simulink model "Bidirectional_Charger_for_EVs"  (R2023a)
settings: Solver=VariableStepAuto  StartTime=0.0  StopTime=0.5  RelTol=1e-3
values from neighbouring files (symbols this model uses):
  fsw = 120e3    (= 120000)    [parametreler_DAB.m]
  Kp = sqrt(fsw*L)    [parametreler_DAB.m]
  L = 20e-6    (= 2e-05)    [parametreler_DAB.m]
  Tsim = tsw    (= 4.16666666667e-06)    [parametreler_DAB.m]
  tsw = 1/2/fsw    (= 4.16666666667e-06)    [parametreler_DAB.m]
undefined symbols (not defined in the file or in its folder): Ion, Lithium
libraries: spsIGBTDiodeLib x12, spsVoltageMeasurementLib x9, spsMosfetLib x8, spsSeriesRLCBranchLib x8, spsDiodeLib x6, spsCurrentMeasurementLib x5, slpidlib x3, simulink x3, simulink_extras x2, spsTriangleGeneratorLib x2, spsBatteryLib x1, spsLinearTransformerLib x1
settings Model: Creator=Berkan  LastModifiedBy=mahgo
settings ModelReferenceCC: EnableRefExpFcnMdlSchedulingChecks=on

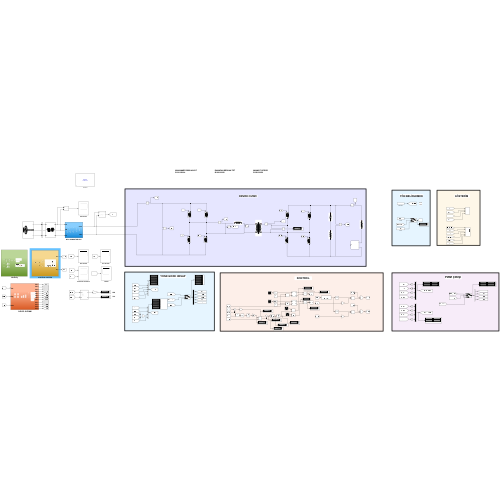
[thumbnail: Simulink's stored preview of the top-level diagram]
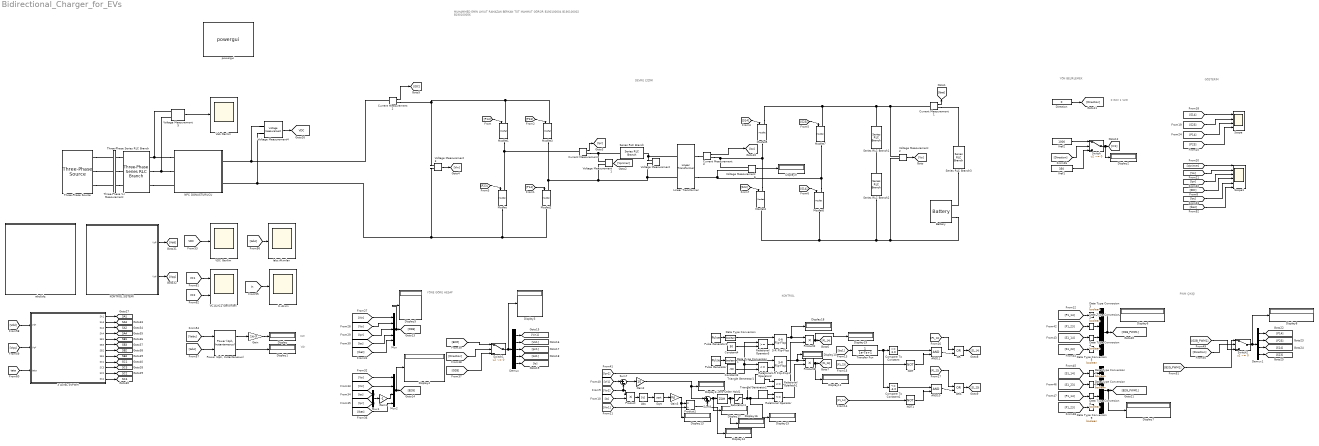
== system Bidirectional_Charger_for_EVs ==
  note: VAr
  note: MUHAMMED EMİN AYKUT RAMAZAN BERKAN TÜT MAHMUT GÖRÜR
      | B190100004 B190100002 B190100056
  note: KW
  note: DEVRE ÇİZİMİ
  note: KONTROL
  note: PWM ÇIKIŞI
  note: 0 G2V
      | 1 V2G
  note: YÖN BELİRLEMEK
  note: GÖSTERİM
  note: YÖNE GÖRE HESAP
  " KONTROL SISTEMI" : Subsystem
  3 LEVEL SVPWM : Subsystem
  AND10 : Logic  IconShape=distinctive  AllPortsSameDT=off  OutDataTypeStr=boolean
  AND11 : Logic  IconShape=distinctive  AllPortsSameDT=off  OutDataTypeStr=boolean
  Abs : Abs  SaturateOnIntegerOverflow=off
  Battery : spsBatteryLib/Battery  BatType=Lithium-Ion  ShowTempParam=off  ThermalPreset=no  ShowAgeParam=off  NomV=350  NomQ=5.4  SOC=0  Batt_Tr=30  PresetModel=on  MaxQ=5.4  MinV=262.5  FullV=407.3955  Dis_rate=2.3478  R=0.64815  Normal_OP=4.8835  expZone="[378.135     0.2653043]"  current=[6.5 13 32.5]  Units=Time  Tci=20  NomT=20  T2=-30  MaxQ2=4.8  FullV2=7.1  Normal_OP2=5.655  expZone2="[6.58           1]"  Rca=0.6  ti=2000  Dp=0  Neq0=0  Tsim=1e6  Ta1=25  Qeol=5.4*0.9  Reol=0.013333*1.2  Char_age=[2.3478, 3]  Dis_age=[2.3478, 10]  N1=1500  N2=10500  N3=1000  N4=1400  Ta2=45  N5=950
  Compare To Constant : simulink/Logic and Bit Operations/Compare To Constant  relop=>=  const=3.0  OutDataTypeStr=boolean
  Compare To Constant1 : simulink/Logic and Bit Operations/Compare To Constant  relop=<=  const=-3.0  OutDataTypeStr=boolean
  Constant3 : Constant  Value=-50
  Constant4 : Constant  Value=50
  Current Measurement{,1..3} (4 alike) : spsCurrentMeasurementLib/Current Measurement  PhasorSimulation=off  OutputType=Complex  PSBequivalent=0
  Data Type Conversion{,1..9} (10 alike) : DataTypeConversion  OutDataTypeStr=boolean  SaturateOnIntegerOverflow=off  RndMeth=Floor
  Demux : Demux  Outputs=5
  Demux1 : Demux
  Direction : Constant  Value=0
  Display{,1..19} (20 alike) : Display
  Gain : Gain  Gain=1e-3
  Gain1 : Gain  Gain=-1
  Gain2 : Gain  Gain=10
  Gain3 : Gain  Gain=Kp
  Iabc Akımları : Scope
  In Akımı : Scope
  Linear Transformer : spsLinearTransformerLib/Linear Transformer  UNITS=SI  NominalPower=[ 250e6 50 ]  winding1=[7.35e+05 4.32 0.45]  winding2=[3.85e+05 4.32 0.45]  ThreeWindings=off  winding3=[3.15e+05 0.7938 6.3169e-05]  RmLm=[1e6 2866]  Measurements=Winding voltages  DataType=on
  Mosfet{,1..7} (8 alike) : spsMosfetLib/Mosfet  Ron=1e-10  Lon=0  Rd=0.01  Vfd=0  IC=0  Rs=1e5  Cs=inf  Measurements=off
  Mux : Mux  Inputs=5
  Mux1 : Mux  Inputs=2
  Mux2 : Mux
  Mux3 : Mux
  Mux4 : Mux
  NOT : Logic  Operator=NOT  IconShape=distinctive  AllPortsSameDT=off  OutDataTypeStr=boolean
  NOT1 : Logic  Operator=NOT  IconShape=distinctive  AllPortsSameDT=off  OutDataTypeStr=boolean
  NPC DONUSTURUCU : Subsystem
  OR : Logic  Operator=OR  IconShape=distinctive  AllPortsSameDT=off  OutDataTypeStr=boolean
  OR1 : Logic  Operator=OR  IconShape=distinctive  AllPortsSameDT=off  OutDataTypeStr=boolean
  "Power (3ph, Instantaneous)" : spsPower3phInstantaneousLib/Power (3ph, Instantaneous)
  Product : Product
  Product1 : Product  Inputs=*/
  Product2 : Product
  Product3 : Product
  Pulse Generator : DiscretePulseGenerator  PulseType=Time based  Period=1/fsw  PulseWidth=10  PhaseDelay=tsw
  Pulse Generator1 : DiscretePulseGenerator  PulseType=Time based  Period=1/fsw  PulseWidth=10  VectorParams1D=off
  Relational Operator : RelationalOperator  Operator=<=  OutDataTypeStr=boolean  RndMeth=Simplest  InputSameDT=off
  Relational Operator1 : RelationalOperator  Operator=<=  OutDataTypeStr=boolean  RndMeth=Simplest  InputSameDT=off
  Relational Operator2 : RelationalOperator  Operator=<=  OutDataTypeStr=boolean  RndMeth=Floor  InputSameDT=off
  Relational Operator3 : RelationalOperator  OutDataTypeStr=boolean  RndMeth=Simplest  InputSameDT=off
  S-R Flip-Flop : simulink_extras/Flip Flops/S-R Flip-Flop  initial_condition=0
  S-R Flip-Flop1 : simulink_extras/Flip Flops/S-R Flip-Flop  initial_condition=0
  Saturation1 : Saturate  LowerLimit=0
  Scope : Scope  NumInputPorts=4
  Scope1 : Scope  NumInputPorts=6
  Series RLC Branch : spsSeriesRLCBranchLib/Series RLC Branch  LConnTagsString=__new0  RConnTagsString=__new0  BranchType=L  Resistance=1  Inductance=L  SetiL0=off  InitialCurrent=0  Capacitance=1e-6  Setx0=off  InitialVoltage=0  Measurements=None
  Series RLC Branch1 : spsSeriesRLCBranchLib/Series RLC Branch  LConnTagsString=__new0  RConnTagsString=__new0  BranchType=C  Resistance=1  Inductance=1e-3  SetiL0=off  InitialCurrent=0  Capacitance=30e-6  Setx0=off  InitialVoltage=0  Measurements=None
  Series RLC Branch2 : spsSeriesRLCBranchLib/Series RLC Branch  LConnTagsString=__new0  RConnTagsString=__new0  BranchType=R  Resistance=3.2e-3  Inductance=1e-3  SetiL0=off  InitialCurrent=0  Capacitance=1e-6  Setx0=off  InitialVoltage=0  Measurements=None
  Series RLC Branch3 : spsSeriesRLCBranchLib/Series RLC Branch  LConnTagsString=__new0  RConnTagsString=__new0  BranchType=R  Resistance=5  Inductance=1e-3  SetiL0=off  InitialCurrent=0  Capacitance=1e-6  Setx0=off  InitialVoltage=0  Measurements=None
  Sqrt : Sqrt
  Sum7 : Sum  Inputs=|+-
  Sum8 : Sum  Inputs=|++
  Switch : Switch  Criteria=u2 ~= 0  SaturateOnIntegerOverflow=off  InputSameDT=off
  Switch1 : Switch  Criteria=u2 ~= 0  SaturateOnIntegerOverflow=off  InputSameDT=off
  Switch2 : Switch  Criteria=u2 ~= 0  SaturateOnIntegerOverflow=off  InputSameDT=off
  Three-Phase Series RLC Branch : spsThreePhaseSeriesRLCBranchLib/Three-Phase Series RLC Branch  LConnTagsString=A|B|C  RConnTagsString=A|B|C  BranchType=RL  Resistance=0.05  Inductance=5e-3  Capacitance=1e-6  Measurements=None
  Three-Phase V-I Measurement : spsThreePhaseVIMeasurementLib/Three-Phase V-I Measurement  VoltageMeasurement=phase-to-ground  SetLabelV=on  LabelV=Vabc  Vpu=off  VpuLL=off  CurrentMeasurement=yes  SetLabelI=on  LabelI=Iabc  Ipu=off  Pbase=100e6  Vbase=500e3  OutputType=Complex  PhasorSimulation=off  PSBequivalent=0
  Three-Phase Source : spsThreePhaseSourceLib/Three-Phase Source  InternalConnection=Yg  VoltagePhases=off  Voltage=380  PhaseAngle=0  Voltage_phases=[25e3 25e3 25e3]/sqrt(3)  PhaseAngles_phases=[0 -120 +120]  Frequency=50  NonIdealSource=on  SpecifyImpedance=off  Resistance=0  Inductance=0  ShortCircuitLevel=100e6  BaseVoltage=380  XRratio=7  BusType=swing  Pref=10e3  Qref=0  Prefabc=[10e3, 10e3, 10e3]  Qrefabc=[0, 0, 0]  Qmin=-inf  Qmax=inf
  Transfer Fcn : TransferFcn  Denominator=[1e-7 1]
  Triangle Generator1 : spsTriangleGeneratorLib/Triangle Generator  Freq=fsw  Phase=0  Ts=Tsim
  Triangle Generator2 : spsTriangleGeneratorLib/Triangle Generator  Freq=fsw  Phase=180  Ts=Tsim
  VC1&VC2 Gerilimleri : Scope  NumInputPorts=2
  VDC Gerilim : Scope
  Vab Gerilim : Scope
  Voltage Measurement{,1..6} (7 alike) : spsVoltageMeasurementLib/Voltage Measurement  PhasorSimulation=off  OutputType=Complex  PSBequivalent=0
  Vref1 : Constant  Value=350
  Vref2 : Constant  Value=1000
  Zero-Order Hold1 : ZeroOrderHold  SampleTime=tsw*2
  abc&dq : Subsystem
  powergui : spspowerguiLib/powergui  Priority=1  SimulationMode=Discrete  SampleTime=1/(fsw)  frequency=60  Iterations=50  frequencyindice=0  Pbase=100e6  ErrMax=1e-4  UnitsV=kV  UnitsW=MW  buscounter=0  FunctionMessages=off  echomessages=off  EnableUseOfTLC=off  CurrentSourceSwitches=off  DisableSnubberDevices=off  DisableRonSwitches=off  DisableVfSwitches=off  DisplayEquations=off  AutomaticDiscreteSolvers=off  SolverType=Tustin/Backward Euler (TBE)  Interpol=off  ExternalGateDelay=off  methode=off  Ts=100  x0status=blocks  SPID=on  SwTol=0  HookPort=off  NonlinearTolerance=1e-4  nMaxIteration=100  ContinueOnMaxIteration=off  RestoreLinks=warning  ResistiveCurrentMeasurement=off  Frange=[0:2:500]  Ylog=off  Xlog=on  ShowGrid=off  save=off  variable=ZData  structure=0  ZoomFFT=off  StartTime=0.0  cycles=1  DisplayStyle=1  fundamental=60  FreqAxis=off  MaxFrequency=1000  frequencyindicesteady=1  RmsSteady=1  display=off
  tag scope: SA1=global, SA2=global, SA3=global, SA4=global, SB1=global, SB2=global, SB3=global, SB4=global, SC1=global, SC2=global, SC3=global, SC4=global, VDC=global
  wires:
  [teta] -> 3 LEVEL SVPWM/3(teta)
  [VC2] -> VC1&VC2 Gerilimleri/2
  [VC1] -> VC1&VC2 Gerilimleri/1
  3 LEVEL SVPWM/7(SB2) -> [SB2]
  [Iabc] -> "Power (3ph, Instantaneous)"/2
  3 LEVEL SVPWM/9(SC1) -> [SC1]
  [In] -> In Akımı/1
  3 LEVEL SVPWM/6(SB3) -> [SB3]
  Voltage Measurement5/1 -> Vab Gerilim/1
  [Vabc] -> "Power (3ph, Instantaneous)"/1
  3 LEVEL SVPWM/10(SC3) -> [SC3]
  3 LEVEL SVPWM/2(SA3) -> [SA3]
  3 LEVEL SVPWM/12(SC4) -> [SC4]
  3 LEVEL SVPWM/11(SC2) -> [SC2]
  3 LEVEL SVPWM/4(SA4) -> [SA4]
  3 LEVEL SVPWM/8(SB4) -> [SB4]
  3 LEVEL SVPWM/1(SA1) -> [SA1]
  [VDC] -> VDC Gerilim/1
  "Power (3ph, Instantaneous)"/1 -> Gain/1
  3 LEVEL SVPWM/3(SA2) -> [SA2]
  [Iabc] -> Iabc Akımları/1
  " KONTROL SISTEMI"/2(Vq*) -> [Vqq]
  " KONTROL SISTEMI"/1(Vd*) -> [Vdd]
  [Vdd] -> 3 LEVEL SVPWM/1(Vd*)
  "Power (3ph, Instantaneous)"/2 -> Display1/1
  3 LEVEL SVPWM/5(SB1) -> [SB1]
  Gain/1 -> Display/1
  [Vqq] -> 3 LEVEL SVPWM/2(Vq*)
  Voltage Measurement4/1 -> [VDC]
  [G2B_PWM1] -> Switch2/3
  Product2/1 -> Display19/1, [P1_14]
  [Ipr] -> Mux/3
  Mux1/1 -> Gain1/1
  Data Type Conversion5/1 -> Mux3/4
  Switch1/1 -> Display3/1, Demux/1
  Sum7/1 -> Gain2/1
  Current Measurement3/1 -> [Isc]
  [Vin] -> Mux/1
  Demux/5 -> [Io]
  [B2G_PWM1] -> Switch2/1
  Triangle Generator1/1 -> Relational Operator1/1
  Voltage Measurement6/1 -> Display9/1
  [Ipr1] -> Relational Operator3/1, Relational Operator2/1
  Demux1/1 -> [P14]
  Vref1/1 -> Switch/3
  [B2G] -> Switch1/1
  Data Type Conversion7/1 -> Mux4/1
  NOT/1 -> AND11/2
  [P1_14] -> Data Type Conversion3/1
  [Ibat] -> Mux/5
  Voltage Measurement3/1 -> [Vin]
  Gain1/1 -> Mux2/3
  Demux/4 -> [Isc1]
  Sqrt/1 -> Gain3/1
  S-R Flip-Flop1/1 -> Display10/1, Product3/1
  [P23] -> Scope/4
  [Vo] -> Mux2/1
  [Isc] -> Scope1/5
  [Ibat] -> Scope1/6
  [S14] -> Mosfet5/1
  Switch/1 -> Display2/1, [Vr1]
  [G2B] -> Switch1/3
  Mux4/1 -> Display7/1, [B2G_PWM1]
  Data Type Conversion6/1 -> Mux4/2
  Demux1/3 -> [S14]
  Data Type Conversion4/1 -> Mux3/3
  Demux/3 -> [Ipr1]
  [Vprimer] -> Scope1/1
  Direction/1 -> [Direction]
  [IDC] -> Scope1/4
  Voltage Measurement1/1 -> [Vprimer]
  [P1_23] -> Data Type Conversion2/1
  Data Type Conversion9/1 -> Mux4/4
  Data Type Conversion2/1 -> Mux3/2
  [P1_23] -> OR1/1
  Data Type Conversion3/1 -> Mux3/1
  Product1/1 -> Display14/1, Sum8/2
  Switch2/1 -> Display8/1, Demux1/1
  [Direction] -> Switch1/2
  [S1_23] -> Data Type Conversion6/1
  Mux3/1 -> Display6/1, [G2B_PWM1]
  Demux1/2 -> [P23]
  Mux/1 -> Display5/1, [G2B]
  [S1_23] -> Data Type Conversion5/1
  Data Type Conversion8/1 -> Mux4/3
  Data Type Conversion1/1 -> S-R Flip-Flop1/1
  [P14] -> Mosfet2/1
  [Ipr] -> Mux1/2
  [S1_14] -> Data Type Conversion4/1
  [Isc] -> Mux/4
  [P1_23] -> Data Type Conversion9/1
  [Direction] -> Switch/2
  Current Measurement1/1 -> [Ibat]
  [P1_14] -> Data Type Conversion8/1
  AND10/1 -> OR1/2
  Vref2/1 -> Switch/1
  Sum8/1 -> Display17/1, Zero-Order Hold1/1
  Saturation1/1 -> Display15/1, Relational Operator/2, Relational Operator1/2
  [Isc] -> Mux1/1
  Product/1 -> Abs/1
  [Vo] -> Mux/2
  [Isc1] -> Transfer Fcn/1
  [S14] -> Scope/1
  [P1_23] -> NOT/1
  Compare To Constant1/1 -> AND10/1
  OR1/1 -> [S1_23]
  Zero-Order Hold1/1 -> Display16/1, Saturation1/1
  Triangle Generator2/1 -> Relational Operator/1
  Gain3/1 -> Display13/1, Product1/1
  Compare To Constant/1 -> AND11/1
  [P23] -> Mosfet3/1
  [P1_14] -> OR/1
  Demux/2 -> [Vo1]
  Current Measurement/1 -> [Ipr]
  Pulse Generator1/1 -> Data Type Conversion/1
  [S1_14] -> Data Type Conversion7/1
  Voltage Measurement2/1 -> [Vo]
  [S23] -> Scope/2
  NOT1/1 -> AND10/2
  Relational Operator/1 -> Product3/2
  [Vo1] -> Product/1, Sum7/2
  [P1_14] -> NOT1/1
  [Vin] -> Mux2/2
  Transfer Fcn/1 -> Compare To Constant1/1, Compare To Constant/1
  [P14] -> Mosfet1/1
  [P14] -> Scope/3
  [Ibat] -> Mux2/4
  Gain2/1 -> Display12/1, Sum8/1
  [Vo] -> Scope1/2
  [Io] -> Product/2
  [S23] -> Mosfet4/1
  Mux2/1 -> Display4/1, [B2G]
  [S23] -> Mosfet7/1
  Data Type Conversion/1 -> S-R Flip-Flop/1
  [S14] -> Mosfet6/1
  AND11/1 -> OR/2
  Constant4/1 -> Relational Operator3/2
  S-R Flip-Flop/1 -> Display18/1, Product2/1
  [P23] -> Mosfet/1
  [Vin1] -> Product1/2
  Pulse Generator/1 -> Data Type Conversion1/1
  Abs/1 -> Sqrt/1
  Relational Operator1/1 -> Product2/2
  [Vr1] -> Sum7/1
  Current Measurement2/1 -> [IDC]
  Relational Operator2/1 -> S-R Flip-Flop1/2
  [Ipr] -> Scope1/3
  OR/1 -> [S1_14]
  Relational Operator3/1 -> S-R Flip-Flop/2
  Product3/1 -> Display11/1, [P1_23]
  Constant3/1 -> Relational Operator2/2
  Demux/1 -> [Vin1]
  [Direction] -> Switch2/2
  Demux1/4 -> [S23]
  connections:
  Voltage Measurement4/LConn1 -- Current Measurement2/LConn1 -- NPC DONUSTURUCU/RConn1
  NPC DONUSTURUCU/LConn2 -- Three-Phase Series RLC Branch/RConn2 -- Voltage Measurement5/LConn2
  NPC DONUSTURUCU/LConn1 -- Three-Phase Series RLC Branch/RConn1 -- Voltage Measurement5/LConn1
  Voltage Measurement3/LConn2 -- Voltage Measurement4/LConn2 -- NPC DONUSTURUCU/RConn2 -- Mosfet2/RConn1 -- Mosfet/RConn1
  Three-Phase V-I Measurement/RConn1 -- Three-Phase Series RLC Branch/LConn1
  Three-Phase Series RLC Branch/RConn3 -- NPC DONUSTURUCU/LConn3
  Three-Phase Source/RConn1 -- Three-Phase V-I Measurement/LConn1
  Three-Phase Source/RConn2 -- Three-Phase V-I Measurement/LConn2
  Three-Phase V-I Measurement/RConn3 -- Three-Phase Series RLC Branch/LConn3
  Three-Phase V-I Measurement/RConn2 -- Three-Phase Series RLC Branch/LConn2
  Three-Phase Source/RConn3 -- Three-Phase V-I Measurement/LConn3
  Mosfet5/LConn1 -- Voltage Measurement2/LConn1 -- Current Measurement1/LConn1 -- Series RLC Branch1/LConn1 -- Mosfet7/LConn1
  Voltage Measurement1/LConn2 -- Voltage Measurement/LConn2 -- Linear Transformer/LConn2 -- Mosfet3/RConn1 -- Mosfet2/LConn1
  Series RLC Branch2/RConn1 -- Battery/LConn2 -- Voltage Measurement2/LConn2 -- Mosfet4/RConn1 -- Mosfet6/RConn1
  Mosfet6/LConn1 -- Mosfet7/RConn1 -- Linear Transformer/RConn2 -- Voltage Measurement6/LConn2
  Mosfet4/LConn1 -- Mosfet5/RConn1 -- Current Measurement3/RConn1 -- Voltage Measurement6/LConn1
  Mosfet3/LConn1 -- Mosfet1/LConn1 -- Voltage Measurement3/LConn1 -- Current Measurement2/RConn1
  Current Measurement/LConn1 -- Mosfet/LConn1 -- Mosfet1/RConn1
  Linear Transformer/LConn1 -- Voltage Measurement/LConn1 -- Series RLC Branch/RConn1
  Voltage Measurement1/LConn1 -- Series RLC Branch/LConn1 -- Current Measurement/RConn1
  Linear Transformer/RConn1 -- Current Measurement3/LConn1
  Series RLC Branch2/LConn1 -- Series RLC Branch1/RConn1
  Current Measurement1/RConn1 -- Series RLC Branch3/LConn1
  Series RLC Branch3/RConn1 -- Battery/LConn1

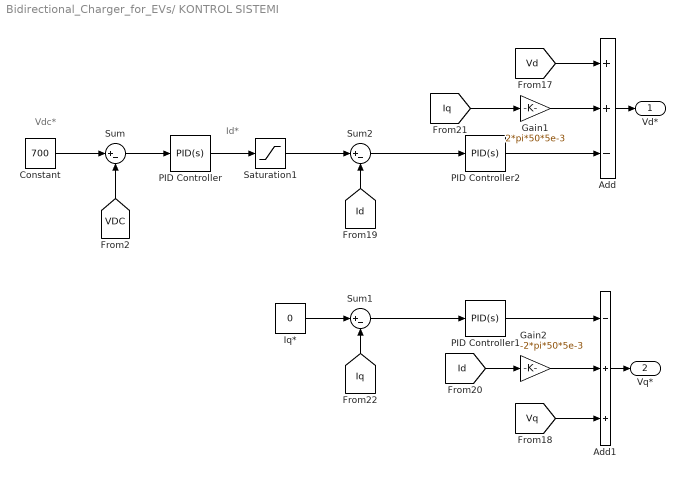
== system Bidirectional_Charger_for_EVs/ KONTROL SISTEMI ==
  note: Vdc*
  note: Id*
  Add : Sum  Inputs=++-
  Add1 : Sum  Inputs=-++
  Constant : Constant  Value=700
  Gain1 : Gain  Gain=2*pi*50*5e-3
  Gain2 : Gain  Gain=-2*pi*50*5e-3
  Iq* : Constant  Value=0
  PID Controller : slpidlib/PID Controller  Controller=PID  Form=Parallel  TimeDomain=Continuous-time  UseExternalTs=off  SampleTime=-1  IntegratorMethod=Forward Euler  FilterMethod=Forward Euler  ControllerParametersSource=internal  P=0.5  I=100  UseKiTs=off  D=0  N=100  UseFilter=on  TunerSelectOption=Transfer Function Based (PID Tuner App)  InitialConditionSource=internal  InitialConditionForIntegrator=0  InitialConditionForFilter=0  DifferentiatorICPrevScaledInput=0  ExternalReset=none  TrackingMode=off  Kt=1  LimitOutput=off  SatLimitsSource=internal  UpperSaturationLimit=inf  LowerSaturationLimit=-inf  LinearizeAsGain=on  AntiWindupMode=none  Kb=1  LimitIntegrator=off  UpperIntegratorSaturationLimit=inf  LowerIntegratorSaturationLimit=-inf  POutMin=[]  POutMax=[]  IOutMin=[]  IOutMax=[]  DOutMin=[]  DOutMax=[]  NOutMin=[]  NOutMax=[]  SumOutMin=[]  SumOutMax=[]  SaturationOutMin=[]  SaturationOutMax=[]  PParamMin=[]  PParamMax=[]  IParamMin=[]  IParamMax=[]  DParamMin=[]  DParamMax=[]  NParamMin=[]  NParamMax=[]  KbParamMin=[]  KbParamMax=[]  KtParamMin=[]  KtParamMax=[]  KbOutMin=[]  KbOutMax=[]  KtOutMin=[]  KtOutMax=[]  IntegratorOutMin=[]  IntegratorOutMax=[]  FilterOutMin=[]  FilterOutMax=[]  SumI1OutMin=[]  SumI1OutMax=[]  SumI2OutMin=[]  SumI2OutMax=[]  SumI3OutMin=[]  SumI3OutMax=[]  SumI4OutMin=[]  SumI4OutMax=[]  SumDOutMin=[]  SumDOutMax=[]  DifferentiatorOutMin=[]  DifferentiatorOutMax=[]  FilterDiffOutCoefMin=[]  FilterDiffOutCoefMax=[]  ReciprocalOutMin=[]  ReciprocalOutMax=[]  SumDenOutMin=[]  SumDenOutMax=[]  SumNumOutMin=[]  SumNumOutMax=[]  DivideOutMin=[]  DivideOutMax=[]  UdiffTsProdOutMin=[]  UdiffTsProdOutMax=[]  NTsProdOutMin=[]  NTsProdOutMax=[]  UintegralTsProdOutMin=[]  UintegralTsProdOutMax=[]  UngainTsProdOutMin=[]  UngainTsProdOutMax=[]  ClampingZeroOutDataTypeStr=Inherit: Inherit via back propagation  ClampingZeroOutMin=[]  ClampingZeroOutMax=[]  FilterDenConstantOutDataTypeStr=Inherit: Inherit via back propagation  FilterDenConstantOutMin=[]  FilterDenConstantOutMax=[]  PCopyOutDataTypeStr=Inherit: Inherit via back propagation  PCopyOutMin=[]  PCopyOutMax=[]  NCopyOutDataTypeStr=Inherit: Inherit via back propagation  NCopyOutMin=[]  NCopyOutMax=[]  IntegratorContinuousStateAttributes=''  IntegratorStateMustResolveToSignalObject=off  IntegratorRTWStateStorageClass=Auto  FilterContinuousStateAttributes=''  FilterStateMustResolveToSignalObject=off  FilterRTWStateStorageClass=Auto  ParallelPVariant=InternalParameters  IdealPVariant=Disabled  IVariant=InternalParameters  DVariant=InternalParameters  IntegratorVariant=Continuous  SatVariant=Disabled  AWVariant=Passthrough  PCopyVariant=Disabled  TRVariant=Disabled  FdbkBlocksVariant=Forward  IdealPFdbkVariant=Disabled  SatFdbkVariant=Disabled  DerivativeFilterVariant=ContFilter  NVariant=InternalParameters  NCopyVariant=Disabled  FilterICVariant=InternalICsFilter  IntegratorICVariant=InternalICs  ExternalResetVariant=Disabled  TRSumVariant=Passthrough  SumFdbkVariant=Disabled  SumVariant=Sum_PID  TsampFilterVariant=InternalTs  TsampNgainVariant=Passthrough  TsampIntegralVariant=Disabled_SignalSpec  ExternalSaturationOutDataTypeStr=Inherit: Same as second input
  PID Controller1 : slpidlib/PID Controller  Controller=PID  Form=Parallel  TimeDomain=Continuous-time  UseExternalTs=off  SampleTime=-1  IntegratorMethod=Forward Euler  FilterMethod=Forward Euler  ControllerParametersSource=internal  P=20000  I=2800  UseKiTs=off  D=0  N=100  UseFilter=on  TunerSelectOption=Transfer Function Based (PID Tuner App)  InitialConditionSource=internal  InitialConditionForIntegrator=0  InitialConditionForFilter=0  DifferentiatorICPrevScaledInput=0  ExternalReset=none  TrackingMode=off  Kt=1  LimitOutput=off  SatLimitsSource=internal  UpperSaturationLimit=inf  LowerSaturationLimit=-inf  LinearizeAsGain=on  AntiWindupMode=none  Kb=1  LimitIntegrator=off  UpperIntegratorSaturationLimit=inf  LowerIntegratorSaturationLimit=-inf  POutMin=[]  POutMax=[]  IOutMin=[]  IOutMax=[]  DOutMin=[]  DOutMax=[]  NOutMin=[]  NOutMax=[]  SumOutMin=[]  SumOutMax=[]  SaturationOutMin=[]  SaturationOutMax=[]  PParamMin=[]  PParamMax=[]  IParamMin=[]  IParamMax=[]  DParamMin=[]  DParamMax=[]  NParamMin=[]  NParamMax=[]  KbParamMin=[]  KbParamMax=[]  KtParamMin=[]  KtParamMax=[]  KbOutMin=[]  KbOutMax=[]  KtOutMin=[]  KtOutMax=[]  IntegratorOutMin=[]  IntegratorOutMax=[]  FilterOutMin=[]  FilterOutMax=[]  SumI1OutMin=[]  SumI1OutMax=[]  SumI2OutMin=[]  SumI2OutMax=[]  SumI3OutMin=[]  SumI3OutMax=[]  SumI4OutMin=[]  SumI4OutMax=[]  SumDOutMin=[]  SumDOutMax=[]  DifferentiatorOutMin=[]  DifferentiatorOutMax=[]  FilterDiffOutCoefMin=[]  FilterDiffOutCoefMax=[]  ReciprocalOutMin=[]  ReciprocalOutMax=[]  SumDenOutMin=[]  SumDenOutMax=[]  SumNumOutMin=[]  SumNumOutMax=[]  DivideOutMin=[]  DivideOutMax=[]  UdiffTsProdOutMin=[]  UdiffTsProdOutMax=[]  NTsProdOutMin=[]  NTsProdOutMax=[]  UintegralTsProdOutMin=[]  UintegralTsProdOutMax=[]  UngainTsProdOutMin=[]  UngainTsProdOutMax=[]  ClampingZeroOutDataTypeStr=Inherit: Inherit via back propagation  ClampingZeroOutMin=[]  ClampingZeroOutMax=[]  FilterDenConstantOutDataTypeStr=Inherit: Inherit via back propagation  FilterDenConstantOutMin=[]  FilterDenConstantOutMax=[]  PCopyOutDataTypeStr=Inherit: Inherit via back propagation  PCopyOutMin=[]  PCopyOutMax=[]  NCopyOutDataTypeStr=Inherit: Inherit via back propagation  NCopyOutMin=[]  NCopyOutMax=[]  IntegratorContinuousStateAttributes=''  IntegratorStateMustResolveToSignalObject=off  IntegratorRTWStateStorageClass=Auto  FilterContinuousStateAttributes=''  FilterStateMustResolveToSignalObject=off  FilterRTWStateStorageClass=Auto  ParallelPVariant=InternalParameters  IdealPVariant=Disabled  IVariant=InternalParameters  DVariant=InternalParameters  IntegratorVariant=Continuous  SatVariant=Disabled  AWVariant=Passthrough  PCopyVariant=Disabled  TRVariant=Disabled  FdbkBlocksVariant=Forward  IdealPFdbkVariant=Disabled  SatFdbkVariant=Disabled  DerivativeFilterVariant=ContFilter  NVariant=InternalParameters  NCopyVariant=Disabled  FilterICVariant=InternalICsFilter  IntegratorICVariant=InternalICs  ExternalResetVariant=Disabled  TRSumVariant=Passthrough  SumFdbkVariant=Disabled  SumVariant=Sum_PID  TsampFilterVariant=InternalTs  TsampNgainVariant=Passthrough  TsampIntegralVariant=Disabled_SignalSpec  ExternalSaturationOutDataTypeStr=Inherit: Same as second input
  PID Controller2 : slpidlib/PID Controller  Controller=PID  Form=Parallel  TimeDomain=Continuous-time  UseExternalTs=off  SampleTime=-1  IntegratorMethod=Forward Euler  FilterMethod=Forward Euler  ControllerParametersSource=internal  P=20000  I=2800  UseKiTs=off  D=0  N=100  UseFilter=on  TunerSelectOption=Transfer Function Based (PID Tuner App)  InitialConditionSource=internal  InitialConditionForIntegrator=0  InitialConditionForFilter=0  DifferentiatorICPrevScaledInput=0  ExternalReset=none  TrackingMode=off  Kt=1  LimitOutput=off  SatLimitsSource=internal  UpperSaturationLimit=inf  LowerSaturationLimit=-inf  LinearizeAsGain=on  AntiWindupMode=none  Kb=1  LimitIntegrator=off  UpperIntegratorSaturationLimit=inf  LowerIntegratorSaturationLimit=-inf  POutMin=[]  POutMax=[]  IOutMin=[]  IOutMax=[]  DOutMin=[]  DOutMax=[]  NOutMin=[]  NOutMax=[]  SumOutMin=[]  SumOutMax=[]  SaturationOutMin=[]  SaturationOutMax=[]  PParamMin=[]  PParamMax=[]  IParamMin=[]  IParamMax=[]  DParamMin=[]  DParamMax=[]  NParamMin=[]  NParamMax=[]  KbParamMin=[]  KbParamMax=[]  KtParamMin=[]  KtParamMax=[]  KbOutMin=[]  KbOutMax=[]  KtOutMin=[]  KtOutMax=[]  IntegratorOutMin=[]  IntegratorOutMax=[]  FilterOutMin=[]  FilterOutMax=[]  SumI1OutMin=[]  SumI1OutMax=[]  SumI2OutMin=[]  SumI2OutMax=[]  SumI3OutMin=[]  SumI3OutMax=[]  SumI4OutMin=[]  SumI4OutMax=[]  SumDOutMin=[]  SumDOutMax=[]  DifferentiatorOutMin=[]  DifferentiatorOutMax=[]  FilterDiffOutCoefMin=[]  FilterDiffOutCoefMax=[]  ReciprocalOutMin=[]  ReciprocalOutMax=[]  SumDenOutMin=[]  SumDenOutMax=[]  SumNumOutMin=[]  SumNumOutMax=[]  DivideOutMin=[]  DivideOutMax=[]  UdiffTsProdOutMin=[]  UdiffTsProdOutMax=[]  NTsProdOutMin=[]  NTsProdOutMax=[]  UintegralTsProdOutMin=[]  UintegralTsProdOutMax=[]  UngainTsProdOutMin=[]  UngainTsProdOutMax=[]  ClampingZeroOutDataTypeStr=Inherit: Inherit via back propagation  ClampingZeroOutMin=[]  ClampingZeroOutMax=[]  FilterDenConstantOutDataTypeStr=Inherit: Inherit via back propagation  FilterDenConstantOutMin=[]  FilterDenConstantOutMax=[]  PCopyOutDataTypeStr=Inherit: Inherit via back propagation  PCopyOutMin=[]  PCopyOutMax=[]  NCopyOutDataTypeStr=Inherit: Inherit via back propagation  NCopyOutMin=[]  NCopyOutMax=[]  IntegratorContinuousStateAttributes=''  IntegratorStateMustResolveToSignalObject=off  IntegratorRTWStateStorageClass=Auto  FilterContinuousStateAttributes=''  FilterStateMustResolveToSignalObject=off  FilterRTWStateStorageClass=Auto  ParallelPVariant=InternalParameters  IdealPVariant=Disabled  IVariant=InternalParameters  DVariant=InternalParameters  IntegratorVariant=Continuous  SatVariant=Disabled  AWVariant=Passthrough  PCopyVariant=Disabled  TRVariant=Disabled  FdbkBlocksVariant=Forward  IdealPFdbkVariant=Disabled  SatFdbkVariant=Disabled  DerivativeFilterVariant=ContFilter  NVariant=InternalParameters  NCopyVariant=Disabled  FilterICVariant=InternalICsFilter  IntegratorICVariant=InternalICs  ExternalResetVariant=Disabled  TRSumVariant=Passthrough  SumFdbkVariant=Disabled  SumVariant=Sum_PID  TsampFilterVariant=InternalTs  TsampNgainVariant=Passthrough  TsampIntegralVariant=Disabled_SignalSpec  ExternalSaturationOutDataTypeStr=Inherit: Same as second input
  Saturation1 : Saturate  UpperLimit=45  LowerLimit=-45
  Sum : Sum  Inputs=|+-
  Sum1 : Sum  Inputs=|+-
  Sum2 : Sum  Inputs=|+-
  Vd* : Outport
  Vq* : Outport  Port=2
  wires:
  PID Controller1/1 -> Add1/1
  Gain2/1 -> Add1/2
  Sum2/1 -> PID Controller2/1
  Add/1 -> Vd*/1
  Sum1/1 -> PID Controller1/1
  Constant/1 -> Sum/1
  Gain1/1 -> Add/2
  [VDC] -> Sum/2
  [Id] -> Sum2/2
  [Id] -> Gain2/1
  [Iq] -> Gain1/1
  [Vd] -> Add/1
  [Vq] -> Add1/3
  PID Controller2/1 -> Add/3
  Add1/1 -> Vq*/1
  Sum/1 -> PID Controller/1
  PID Controller/1 -> Saturation1/1
  Saturation1/1 -> Sum2/1
  [Iq] -> Sum1/2
  Iq*/1 -> Sum1/1

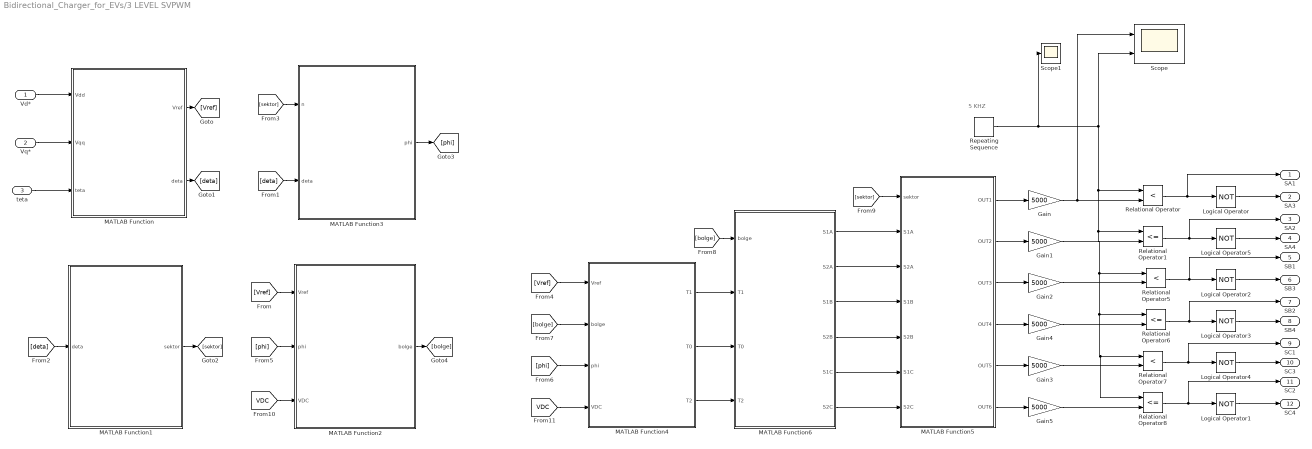
== system Bidirectional_Charger_for_EVs/3 LEVEL SVPWM ==
  note: 5 KHZ
  Vd* : Inport
  Vq* : Inport  Port=2
  teta : Inport  Port=3
  Gain{,1..5} (6 alike) : Gain  Gain=5000
  Logical Operator{,1..5} (6 alike) : Logic  Operator=NOT  AllPortsSameDT=off  OutDataTypeStr=boolean
  MATLAB Function : MATLAB Function  TreatAsAtomicUnit=on
  MATLAB Function1 : MATLAB Function  TreatAsAtomicUnit=on
  MATLAB Function2 : MATLAB Function  TreatAsAtomicUnit=on
  MATLAB Function3 : MATLAB Function  TreatAsAtomicUnit=on
  MATLAB Function4 : MATLAB Function  TreatAsAtomicUnit=on
  MATLAB Function5 : MATLAB Function  TreatAsAtomicUnit=on
  MATLAB Function6 : MATLAB Function  TreatAsAtomicUnit=on
  Relational Operator : RelationalOperator  Operator=<  OutDataTypeStr=boolean  RndMeth=Simplest  InputSameDT=off
  Relational Operator1 : RelationalOperator  Operator=<=  OutDataTypeStr=boolean  RndMeth=Simplest  InputSameDT=off
  Relational Operator5 : RelationalOperator  Operator=<  OutDataTypeStr=boolean  RndMeth=Simplest  InputSameDT=off
  Relational Operator6 : RelationalOperator  Operator=<=  OutDataTypeStr=boolean  RndMeth=Simplest  InputSameDT=off
  Relational Operator7 : RelationalOperator  Operator=<  OutDataTypeStr=boolean  RndMeth=Simplest  InputSameDT=off
  Relational Operator8 : RelationalOperator  Operator=<=  OutDataTypeStr=boolean  RndMeth=Simplest  InputSameDT=off
  Repeating Sequence : simulink/Sources/Repeating Sequence  rep_seq_t=[0 1e-4 2e-4]  rep_seq_y=[0 0.5 0]
  Scope : Scope  NumInputPorts=2
  Scope1 : Scope
  SA1 : Outport
  SA3 : Outport  Port=2
  SA2 : Outport  Port=3
  SA4 : Outport  Port=4
  SB1 : Outport  Port=5
  SB3 : Outport  Port=6
  SB2 : Outport  Port=7
  SB4 : Outport  Port=8
  SC1 : Outport  Port=9
  SC3 : Outport  Port=10
  SC2 : Outport  Port=11
  SC4 : Outport  Port=12
  wires:
  MATLAB Function4/1(T1) -> MATLAB Function6/2(T1)
  MATLAB Function4/3(T2) -> MATLAB Function6/4(T2)
  Repeating Sequence/1 -> Scope1/1, Relational Operator1/1, Relational Operator8/1, Relational Operator7/1, Relational Operator6/1, Relational Operator5/1, Relational Operator/1, Scope/2
  [bolge] -> MATLAB Function6/1(bolge)
  Relational Operator5/1 -> SB1/1, Logical Operator2/1
  [phi] -> MATLAB Function4/3(phi)
  MATLAB Function6/2(S2A) -> MATLAB Function5/3(S2A)
  MATLAB Function2/1(bolge) -> [bolge]
  Relational Operator1/1 -> SA2/1, Logical Operator5/1
  Gain5/1 -> Relational Operator8/2
  Relational Operator/1 -> SA1/1, Logical Operator/1
  MATLAB Function5/5(OUT5) -> Gain3/1
  MATLAB Function5/1(OUT1) -> Gain/1
  MATLAB Function4/2(T0) -> MATLAB Function6/3(T0)
  [bolge] -> MATLAB Function4/2(bolge)
  MATLAB Function6/5(S1C) -> MATLAB Function5/6(S1C)
  MATLAB Function6/4(S2B) -> MATLAB Function5/5(S2B)
  Relational Operator8/1 -> SC2/1, Logical Operator1/1
  [deta] -> MATLAB Function3/2(deta)
  Gain1/1 -> Relational Operator1/2
  MATLAB Function/2(deta) -> [deta]
  MATLAB Function6/1(S1A) -> MATLAB Function5/2(S1A)
  Logical Operator1/1 -> SC4/1
  Gain3/1 -> Relational Operator7/2
  MATLAB Function6/3(S1B) -> MATLAB Function5/4(S1B)
  MATLAB Function6/6(S2C) -> MATLAB Function5/7(S2C)
  Relational Operator6/1 -> SB2/1, Logical Operator3/1
  Relational Operator7/1 -> SC1/1, Logical Operator4/1
  MATLAB Function5/4(OUT4) -> Gain4/1
  Gain/1 -> Scope/1, Relational Operator/2
  MATLAB Function3/1(phi) -> [phi]
  [sektor] -> MATLAB Function3/1(n)
  Gain2/1 -> Relational Operator5/2
  Logical Operator4/1 -> SC3/1
  Gain4/1 -> Relational Operator6/2
  MATLAB Function5/3(OUT3) -> Gain2/1
  MATLAB Function5/2(OUT2) -> Gain1/1
  MATLAB Function5/6(OUT6) -> Gain5/1
  Logical Operator2/1 -> SB3/1
  MATLAB Function/1(Vref) -> [Vref]
  [phi] -> MATLAB Function2/2(phi)
  Logical Operator5/1 -> SA4/1
  [sektor] -> MATLAB Function5/1(sektor)
  [Vref] -> MATLAB Function2/1(Vref)
  [deta] -> MATLAB Function1/1(deta)
  [Vref] -> MATLAB Function4/1(Vref)
  Logical Operator3/1 -> SB4/1
  Logical Operator/1 -> SA3/1
  Vd*/1 -> MATLAB Function/1(Vdd)
  teta/1 -> MATLAB Function/3(teta)
  Vq*/1 -> MATLAB Function/2(Vqq)
  [VDC] -> MATLAB Function2/3(VDC)
  [VDC] -> MATLAB Function4/4(VDC)
  MATLAB Function1/1(sektor) -> [sektor]

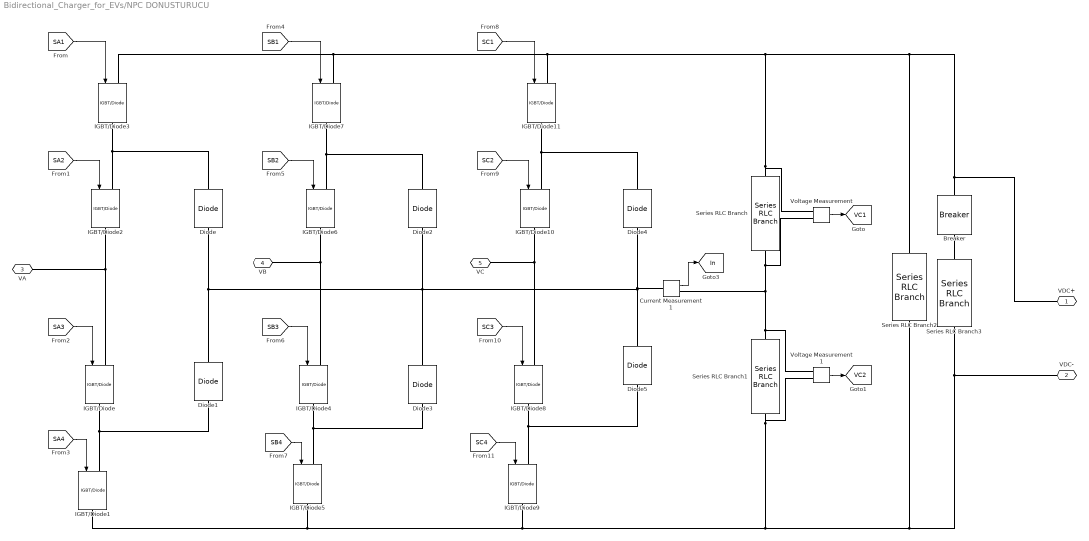
== system Bidirectional_Charger_for_EVs/NPC DONUSTURUCU ==
  Breaker : spsBreakerLib/Breaker  InitialState=0  SwitchingTimes=[0.3]  External=off  BreakerResistance=0.01  SnubberResistance=1e6  SnubberCapacitance=inf  Measurements=None  MoreParameters=on  NoBreakLoop=off
  Current Measurement1 : spsCurrentMeasurementLib/Current Measurement  PhasorSimulation=off  OutputType=Complex  PSBequivalent=0
  Diode{,1..5} (6 alike) : spsDiodeLib/Diode  Ron=0.001  Lon=0  Vf=0.8  IC=0  UseSnubber=0  Rs=500  Cs=250e-9  Measurements=off
  IGBT/Diode{,1..11} (12 alike) : spsIGBTDiodeLib/IGBT//Diode  Ron=1e-3  Rs=1e5  Cs=inf  Measurements=off
  Series RLC Branch : spsSeriesRLCBranchLib/Series RLC Branch  LConnTagsString=__new0  RConnTagsString=__new0  BranchType=C  Resistance=1  Inductance=1e-3  SetiL0=off  InitialCurrent=0  Capacitance=1500e-6  Setx0=on  InitialVoltage=345  Measurements=None
  Series RLC Branch1 : spsSeriesRLCBranchLib/Series RLC Branch  LConnTagsString=__new0  RConnTagsString=__new0  BranchType=C  Resistance=1  Inductance=1e-3  SetiL0=off  InitialCurrent=0  Capacitance=1500e-6  Setx0=on  InitialVoltage=345  Measurements=None
  Series RLC Branch2 : spsSeriesRLCBranchLib/Series RLC Branch  LConnTagsString=__new0  RConnTagsString=__new0  BranchType=R  Resistance=50  Inductance=1e-3  SetiL0=off  InitialCurrent=0  Capacitance=1e-6  Setx0=off  InitialVoltage=0  Measurements=None
  Series RLC Branch3 : spsSeriesRLCBranchLib/Series RLC Branch  LConnTagsString=__new0  RConnTagsString=__new0  BranchType=R  Resistance=50  Inductance=1e-3  SetiL0=off  InitialCurrent=0  Capacitance=1e-6  Setx0=off  InitialVoltage=0  Measurements=None
  Voltage Measurement : spsVoltageMeasurementLib/Voltage Measurement  PhasorSimulation=off  OutputType=Complex  PSBequivalent=0
  Voltage Measurement1 : spsVoltageMeasurementLib/Voltage Measurement  PhasorSimulation=off  OutputType=Complex  PSBequivalent=0
  VDC+ : PMIOPort  Side=Right
  VDC- : PMIOPort  Port=2  Side=Right
  VA : PMIOPort  Port=3  Side=Left
  VB : PMIOPort  Port=4  Side=Left
  VC : PMIOPort  Port=5  Side=Left
  tag scope: In=global, VC1=global, VC2=global
  wires:
  [SA4] -> IGBT/Diode1/1
  [SB2] -> IGBT/Diode6/1
  [SB3] -> IGBT/Diode4/1
  [SC1] -> IGBT/Diode11/1
  [SB4] -> IGBT/Diode5/1
  [SA3] -> IGBT/Diode/1
  [SC4] -> IGBT/Diode9/1
  [SA2] -> IGBT/Diode2/1
  [SB1] -> IGBT/Diode7/1
  [SA1] -> IGBT/Diode3/1
  [SC2] -> IGBT/Diode10/1
  [SC3] -> IGBT/Diode8/1
  Voltage Measurement/1 -> [VC1]
  Voltage Measurement1/1 -> [VC2]
  Current Measurement1/1 -> [In]
  connections:
  IGBT/Diode6/RConn1 -- VB/RConn1 -- IGBT/Diode4/LConn1
  IGBT/Diode1/RConn1 -- IGBT/Diode5/RConn1 -- Voltage Measurement1/LConn2 -- Series RLC Branch1/RConn1 -- VDC-/RConn1 -- Series RLC Branch3/RConn1 -- Series RLC Branch2/RConn1 -- IGBT/Diode9/RConn1
  Diode/LConn1 -- Diode1/RConn1 -- Diode2/LConn1 -- Current Measurement1/LConn1 -- Diode4/LConn1 -- Diode5/RConn1 -- Diode3/RConn1
  IGBT/Diode3/RConn1 -- IGBT/Diode2/LConn1 -- Diode/RConn1
  IGBT/Diode3/LConn1 -- IGBT/Diode7/LConn1 -- VDC+/RConn1 -- Breaker/LConn1 -- Series RLC Branch2/LConn1 -- Voltage Measurement/LConn1 -- Series RLC Branch/LConn1 -- IGBT/Diode11/LConn1
  IGBT/Diode2/RConn1 -- VA/RConn1 -- IGBT/Diode/LConn1
  IGBT/Diode8/RConn1 -- Diode5/LConn1 -- IGBT/Diode9/LConn1
  IGBT/Diode4/RConn1 -- Diode3/LConn1 -- IGBT/Diode5/LConn1
  IGBT/Diode7/RConn1 -- IGBT/Diode6/LConn1 -- Diode2/RConn1
  IGBT/Diode11/RConn1 -- IGBT/Diode10/LConn1 -- Diode4/RConn1
  IGBT/Diode10/RConn1 -- VC/RConn1 -- IGBT/Diode8/LConn1
  IGBT/Diode/RConn1 -- Diode1/LConn1 -- IGBT/Diode1/LConn1
  Breaker/RConn1 -- Series RLC Branch3/LConn1
  Voltage Measurement1/LConn1 -- Current Measurement1/RConn1 -- Voltage Measurement/LConn2 -- Series RLC Branch/RConn1 -- Series RLC Branch1/LConn1

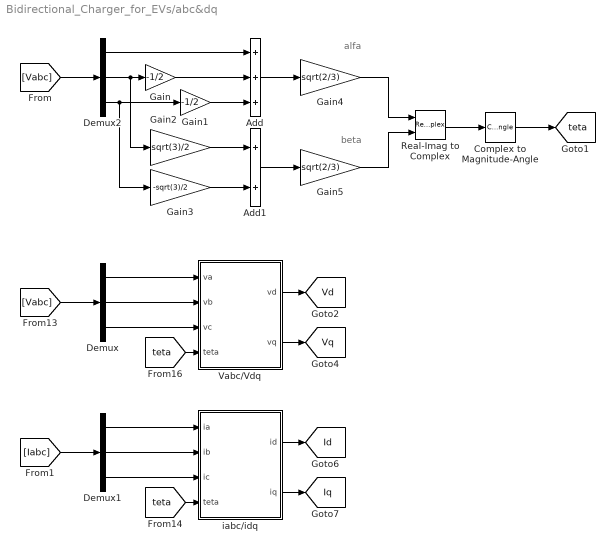
== system Bidirectional_Charger_for_EVs/abc&dq ==
  note: beta
  note: alfa
  Add : Sum  Inputs=+++
  Add1 : Sum
  Complex to Magnitude-Angle : ComplexToMagnitudeAngle  Output=Angle
  Demux : Demux  Outputs=3
  Demux1 : Demux  Outputs=3
  Demux2 : Demux  Outputs=3
  Gain : Gain  Gain=-1/2
  Gain1 : Gain  Gain=-1/2
  Gain2 : Gain  Gain=sqrt(3)/2
  Gain3 : Gain  Gain=-sqrt(3)/2
  Gain4 : Gain  Gain=sqrt(2/3)
  Gain5 : Gain  Gain=sqrt(2/3)
  Real-Imag to Complex : RealImagToComplex
  Vabc/Vdq : MATLAB Function  TreatAsAtomicUnit=on
  iabc/idq : MATLAB Function  TreatAsAtomicUnit=on
  tag scope: Id=global, Iq=global, Vd=global, Vq=global, teta=global
  wires:
  Demux/1 -> Vabc/Vdq/1(va)
  Demux1/1 -> iabc/idq/1(ia)
  Demux1/3 -> iabc/idq/3(ic)
  Demux1/2 -> iabc/idq/2(ib)
  [Iabc] -> Demux1/1
  iabc/idq/1(id) -> [Id]
  Vabc/Vdq/2(vq) -> [Vq]
  Complex to Magnitude-Angle/1 -> [teta]
  Demux/3 -> Vabc/Vdq/3(vc)
  Demux/2 -> Vabc/Vdq/2(vb)
  [Vabc] -> Demux/1
  [teta] -> Vabc/Vdq/4(teta)
  [teta] -> iabc/idq/4(teta)
  iabc/idq/2(iq) -> [Iq]
  Vabc/Vdq/1(vd) -> [Vd]
  Gain1/1 -> Add/3
  Real-Imag to Complex/1 -> Complex to Magnitude-Angle/1
  Gain2/1 -> Add1/1
  Gain3/1 -> Add1/2
  [Vabc] -> Demux2/1
  Add1/1 -> Gain5/1
  Gain/1 -> Add/2
  Add/1 -> Gain4/1
  Gain4/1 -> Real-Imag to Complex/1
  Demux2/3 -> Gain3/1, Gain1/1
  Gain5/1 -> Real-Imag to Complex/2
  Demux2/2 -> Gain2/1, Gain/1
  Demux2/1 -> Add/1

== matlab function Bidirectional_Charger_for_EVs/abc&dq/Vabc//Vdq ==
  data: va input; vd output; vb input; vc input; teta input; vq output
function [vd,vq]= fcn(va,vb,vc,teta)

vd = 2/3*(va*cos(teta)+vb*cos(teta-2*pi/3)+vc*cos(teta+2*pi/3));
vq = -2/3*(va*sin(teta)+vb*sin(teta-2*pi/3)+vc*sin(teta+2*pi/3));

== matlab function Bidirectional_Charger_for_EVs/abc&dq/iabc//idq ==
  data: ia input; id output; ib input; ic input; teta input; iq output
function [id,iq]= fcn(ia,ib,ic,teta)

id = 2/3*(ia*cos(teta)+ib*cos(teta-2*pi/3)+ic*cos(teta+2*pi/3));
iq = -2/3*(ia*sin(teta)+ib*sin(teta-2*pi/3)+ic*sin(teta+2*pi/3));

== matlab function Bidirectional_Charger_for_EVs/3 LEVEL SVPWM/MATLAB Function1 ==
  data: deta input; sektor output
function sektor= Sektor_Belirleme(deta)
sektor=0;
if (deta>=0)  && (deta<pi/3)
    sektor=1;
end
if (deta>=pi/3) && (deta<2*pi/3)
    sektor=2;
end
if (deta>=2*pi/3) && (deta<pi)
    sektor=3;
end
if (deta>=-pi) && (deta<-2*pi/3)
    sektor=4;
end
if (deta>=-2*pi/3) && (deta<-pi/3)
    sektor=5;
end
if (deta>=-pi/3) && (deta<0)
    sektor=6;
end

== matlab function Bidirectional_Charger_for_EVs/3 LEVEL SVPWM/MATLAB Function ==
  data: Vdd input; Vqq input; teta input; Vref output; deta output
function [Vref,deta] = Clarke(Vdd,Vqq,teta)
Valpha=0;
Vbeta=0;
Valpha=Vdd*cos(teta)-Vqq*sin(teta);
Vbeta=Vdd*sin(teta)+Vqq*cos(teta);
deta=atan2(Vbeta,Valpha);
Vref=sqrt(Valpha^2+Vbeta^2);

== matlab function Bidirectional_Charger_for_EVs/3 LEVEL SVPWM/MATLAB Function3 ==
  data: n input; phi output; deta input
function phi = PHI(n,deta)
phi=0;
if (n==1)
    phi=deta;
end

if (n==2)
    phi=deta-pi/3;
end

if (n==3)
    phi=deta-2*pi/3;
end

if (n==4)
    phi=deta+pi;
end

if (n==5)
    phi=2*pi/3+deta;
end

if (n==6)
    phi=pi/3+deta;
end

== matlab function Bidirectional_Charger_for_EVs/3 LEVEL SVPWM/MATLAB Function2 ==
  data: Vref input; bolge output; phi input; VDC input
function bolge = Bolge_Belirleme(Vref,phi,VDC)
bolge=0;
m=Vref/(2/3*VDC);
m1=m*2/sqrt(3)*sin(pi/3-phi);
m2=m*2/sqrt(3)*sin(phi);

if (m1<0.5) && (m2<0.5) && (m1+m2<0.5)
    bolge=1;
end
if (m1<0.5) && (m2<0.5) && (m1+m2>0.5)
    bolge=2;
end
if (m2>0.5)
    bolge=3;
end
if (m1>0.5)
    bolge=4;
end

== matlab function Bidirectional_Charger_for_EVs/3 LEVEL SVPWM/MATLAB Function4 ==
  data: Vref input; T1 output; bolge input; phi input; VDC input; T0 output; T2 output
function [T1,T0,T2] = Anahtarlama_Sureleri(Vref,bolge,phi,VDC)
Ts=1/5000;
T1=0;
T0=0;
T2=0;
m=Vref/(2/3*VDC);
k=2/sqrt(3)*m*Ts;

if (bolge==1)
    T1=2*k*sin(pi/3-phi);
    T0=Ts-2*k*sin(pi/3+phi);
    T2=2*k*sin(phi);
end
if (bolge==2)
    T1=Ts-2*k*sin(phi);
    T0=2*k*sin(pi/3+phi)-Ts;
    T2=Ts-2*k*sin(pi/3-phi);
end
if (bolge==3)
    T1=2*k*sin(phi)-Ts;
    T0=2*k*sin(pi/3-phi);
    T2=2*Ts-2*k*sin(pi/3+phi);
end
if (bolge==4)
    T1=2*Ts-2*k*sin(pi/3+phi);
    T0=2*k*sin(phi);
    T2=2*k*sin(pi/3-phi)-Ts;
end

== matlab function Bidirectional_Charger_for_EVs/3 LEVEL SVPWM/MATLAB Function5 ==
  data: sektor input; OUT1 output; S1A input; S2A input; S1B input; S2B input; S1C input; S2C input; OUT2 output; OUT3 output; OUT4 output; OUT5 output; OUT6 output
function [OUT1,OUT2,OUT3,OUT4,OUT5,OUT6] =Referans_Sinyal(sektor,S1A,S2A,S1B,S2B,S1C,S2C)
Ts=1/5000;
OUT1=0;
OUT2=0;
OUT3=0;
OUT4=0;
OUT5=0;
OUT6=0;
 if (sektor==1)
     OUT1=S1A;
     OUT2=S2A;
     OUT3=S1B;
     OUT4=S2B;
     OUT5=S1C;
     OUT6=S2C;
 end
  if (sektor==2)
     OUT1=Ts/2-S2B;
     OUT2=Ts/2-S1B;
     OUT3=Ts/2-S2C;
     OUT4=Ts/2-S1C;
     OUT5=Ts/2-S2A;
     OUT6=Ts/2-S1A;
  end
  if (sektor==3)
     OUT1=S1C;
     OUT2=S2C;
     OUT3=S1A;
     OUT4=S2A;
     OUT5=S1B;
     OUT6=S2B;
  end
  if (sektor==4)
     OUT1=Ts/2-S2A;
     OUT2=Ts/2-S1A;
     OUT3=Ts/2-S2B;
     OUT4=Ts/2-S1B;
     OUT5=Ts/2-S2C;
     OUT6=Ts/2-S1C;
  end
  if (sektor==5)
     OUT1=S1B;
     OUT2=S2B;
     OUT3=S1C;
     OUT4=S2C;
     OUT5=S1A;
     OUT6=S2A;
  end
  if (sektor==6)
     OUT1=Ts/2-S2C;
     OUT2=Ts/2-S1C;
     OUT3=Ts/2-S2A;
     OUT4=Ts/2-S1A;
     OUT5=Ts/2-S2B;
     OUT6=Ts/2-S1B;
  end

== matlab function Bidirectional_Charger_for_EVs/3 LEVEL SVPWM/MATLAB Function6 ==
  data: bolge input; S1A output; T1 input; T0 input; T2 input; S2A output; S1B output; S2B output; S1C output; S2C output
function [S1A,S2A,S1B,S2B,S1C,S2C]=Anahtarlama_dizilimleri(bolge,T1,T0,T2)
Ts=1/5000;
S1A=0;
S2A=0;
S1B=0;
S2B=0;
S1C=0;
S2C=0;
 if (bolge==1)
     S1A=T2/4+T1/4;
     S2A=Ts/2;
     S1B=T2/4;
     S2B=Ts/2-T1/4;
     S1C=0;
     S2C=Ts/2-T1/4-T2/4;
 end
 if (bolge==2)
     S1A=T2/4+T1/4+T0/2;
     S2A=Ts/2;
     S1B=T2/4;
     S2B=Ts/2-T1/4;
     S1C=0;
     S2C=T1/4+T2/4;
 end
 if (bolge==3)
     S1A=Ts/2-T2/4;
     S2A=Ts/2;
     S1B=T2/4+T1/2;
     S2B=Ts/2;
     S1C=0;
     S2C=T2/4;
 end
 if (bolge==4)
     S1A=Ts/2-T1/4;
     S2A=Ts/2;
     S1B=0;
     S2B=T1/4+T0/2;
     S1C=0;
     S2C=T1/4;
 end
